simulink library "lib_controls"  (Simulink 7.9)
settings: Solver=ode45  SolverMode=SingleTasking  StartTime=0.0  StopTime=10.0  RelTol=1e-3
undefined symbols (not defined in the file or in its folder): amb_tmp, cs_charge_deplete_bool, cs_charge_pwr, cs_charge_trq, cs_clt_tmp, cs_decel_fc_off, cs_decel_regen_threshold, cs_dl_assist_trq_threshold, cs_dl_regen_trq_threshold, cs_electric_decel_spd, cs_electric_launch_spd, cs_electric_launch_spd_hi, cs_electric_launch_spd_lo, cs_eng_min_spd, cs_eng_on_soc, cs_fc_init_state, cs_fc_max_pwr_frac, cs_fc_min_pwr_frac, cs_fc_on, cs_fc_pwr_opt, cs_fc_spd_opt, cs_fuzzy_fuel_mode, cs_hi_soc, cs_hi_trq_frac, cs_lo_soc, cs_lo_trq_frac, cs_max_gc_spd, cs_max_pwr, cs_max_pwr_fall_rate, cs_max_pwr_rise_rate, cs_mc_assist_max_frac, cs_mc_assist_min_frac, cs_mc_assist_slope, cs_mc_regen_max_frac, cs_mc_regen_min_frac, cs_mc_regen_slope, cs_mean_eff, cs_mean_eff_bool, cs_min_gc_spd, cs_min_off_time, cs_min_pwr, cs_min_trq_frac, cs_mph_avg_time, cs_off_trq_frac, cs_plot_output, cs_pwr, cs_regen_avg_time, cs_scale_factor, cs_shutoff, cs_soc_range, cs_spd, cs_target_soc, cs_trq_to_soc_factor, cvt_locus_pwr, cvt_locus_spd, cyc_mph, enable_sim_stop_distance, enable_sim_stop_max_spd, enable_sim_stop_speed, enable_sim_stop_time ... (+110)
libraries: lib_controls x124, simulink3 x13, simulink x5, lib_etc x1
(part 2 of 17)

== system lib_controls/<vc> insight ==
  Ground : Ground
  Relational Operator : RelationalOperator  Operator=~=  InputSameDT=on
  Sum : Sum  Inputs=-+  SaturateOnIntegerOverflow=on  InputSameDT=on  OutDataTypeStr=Inherit: Same as first input
  braking strategy : lib_controls/SubSystem/braking strategy
  config traction control : Subsystem  BlockChoice=traction control 2 axle
      settings: AttributesFormatString=%<BlockChoice>  TemplateBlock=lib_controls/SubSystem/config traction control  MemberBlocks=traction control 2 axle,traction control J2452 2 axle
  engine on (insight) : Subsystem
  front and rear brake controller (achievable) : lib_controls/SubSystem/front and rear brake controller (achievable)
  motor controller logic : Subsystem
  parallel clutch control : Subsystem
  pre-TX parallel gearbox control : Subsystem
  sim stop subsystem : lib_controls/SubSystem/sim stop subsystem
  clutch state : Outport
  tag scope: F_front_brake=global, F_front_brake_req=global, F_rear_brake=global, F_rear_brake_req=global, F_req_limited=global, P_mc_in_r=global, clutch_state=global, engine_on=global, front_traction_ratio=global, gear_number=global, gear_ratio=global, key_on=global, shifting=global, slip_limited=global, spd_command=global, v_req_limited=global, wt_front_axle=global, wt_rear_axle=global
  wires:
  [eta_gb] -> pre-TX parallel gearbox control/3(prev. Pout/Pin)
  [w_gb_out] -> pre-TX parallel gearbox control/2(gb_spd_out_r)
  [T_gb_out] -> pre-TX parallel gearbox control/1(gb_trq_out_r)
  [slip_limited] -> pre-TX parallel gearbox control/4(tires are at traction limit)
  motor controller logic/1(req'd input power (W)1) -> [P_mc_in_r]
  [w_mc_out_r] -> motor controller logic/3(req'd output spd (rad/s))
  [P_mc_in_1lim] -> motor controller logic/2(req'd input power (W))
  [bus_voltage] -> motor controller logic/1(bus voltage)
  front and rear brake controller (achievable)/2 -> [F_rear_brake]
  [F_max_rear_brake] -> front and rear brake controller (achievable)/5
  [F_max_front_brake] -> front and rear brake controller (achievable)/4
  [w_wheel_ach] -> front and rear brake controller (achievable)/3
  [F_drivetrain_ach] -> front and rear brake controller (achievable)/2
  front and rear brake controller (achievable)/1 -> [F_front_brake]
  [v_ave_req] -> braking strategy/1, engine on (insight)/4(v_ave_req), config traction control/1(time-average vehicle speed  req'd (m/s))
  config traction control/3(weight on front axle (N)) -> [wt_front_axle]
  [v_prev] -> config traction control/2(vehicle speed at beginning of time  step (m/s))
  braking strategy/1 -> [F_front_brake_req]
  [F_req] -> front and rear brake controller (achievable)/1, Relational Operator/2, config traction control/3(total tractive force req'd (N))
  config traction control/1(req'd force (N)) -> braking strategy/2, Sum/2, Relational Operator/1
  braking strategy/2 -> Sum/1, [F_rear_brake_req]
  Sum/1 -> [F_req_limited]
  Relational Operator/1 -> [slip_limited]
  config traction control/2(req'd speed (m/s)) -> [v_req_limited]
  [shifting] -> motor controller logic/4(shifting)
  parallel clutch control/1(clutch state) -> [clutch_state], clutch state/1, engine on (insight)/5(clutch state)
  engine on (insight)/1(engine on) -> [engine_on], parallel clutch control/4(engine on)
  [w_cl_out] -> parallel clutch control/3(gb_spd_in_r), engine on (insight)/2(spd_clutch_out)
  engine on (insight)/2(spd command  (rad/s)) -> [spd_command]
  [fc_spd_out_r] -> engine on (insight)/3(fc_spd_out_r)
  engine on (insight)/3(key on) -> [key_on]
  [T_cl_out] -> parallel clutch control/2(gb_trq_in_r), engine on (insight)/1(trq_clutch_out)
  [shifting] -> parallel clutch control/1(shifting)
  pre-TX parallel gearbox control/3("shifting, out") -> [shifting]
  pre-TX parallel gearbox control/2("gear ratio, out") -> [gear_ratio]
  pre-TX parallel gearbox control/1("gear number, out") -> [gear_number]
  config traction control/4(weight on rear axle (N)) -> [wt_rear_axle]
  config traction control/5(front/total  traction ratio) -> [front_traction_ratio]
  Ground/1 -> front and rear brake controller (achievable)/6

== system lib_controls/<vc> par ==
  note: force
      | required (N)
  Ground : Ground
  Relational Operator : RelationalOperator  Operator=~=  InputSameDT=on
  Sum : Sum  Inputs=-+  SaturateOnIntegerOverflow=on  InputSameDT=on  OutDataTypeStr=Inherit: Same as first input
  braking strategy : lib_controls/SubSystem/braking strategy
  config traction control : Subsystem  BlockChoice=traction control 2 axle
      settings: AttributesFormatString=%<BlockChoice>  TemplateBlock=lib_controls/SubSystem/config traction control  MemberBlocks=traction control 2 axle,traction control J2452 2 axle
  engine on (parallel hybrid) : Subsystem
  front and rear brake controller (achievable) : lib_controls/SubSystem/front and rear brake controller (achievable)
  motor controller logic : Subsystem
  parallel clutch control : Subsystem
  pre-TX parallel gearbox control : Subsystem
  sim stop subsystem : lib_controls/SubSystem/sim stop subsystem
  clutch state : Outport
  tag scope: F_front_brake=global, F_front_brake_req=global, F_rear_brake=global, F_rear_brake_req=global, F_req_limited=global, P_mc_in_r=global, clutch_state=global, engine_on=global, front_traction_ratio=global, gear_number=global, gear_ratio=global, key_on=global, shifting=global, slip_limited=global, spd_command=global, v_req_limited=global, wt_front_axle=global, wt_rear_axle=global
  wires:
  [bus_voltage] -> motor controller logic/1(bus voltage)
  [P_mc_in_1lim] -> motor controller logic/2(req'd input power (W))
  [w_mc_out_r] -> motor controller logic/3(req'd output spd (rad/s))
  motor controller logic/1(req'd input power (W)1) -> [P_mc_in_r]
  [shifting] -> motor controller logic/4(shifting)
  [slip_limited] -> pre-TX parallel gearbox control/4(tires are at traction limit)
  [T_gb_out] -> pre-TX parallel gearbox control/1(gb_trq_out_r)
  [w_gb_out] -> pre-TX parallel gearbox control/2(gb_spd_out_r)
  [eta_gb] -> pre-TX parallel gearbox control/3(prev. Pout/Pin)
  engine on (parallel hybrid)/3(key on) -> [key_on]
  [fc_spd_out_r] -> engine on (parallel hybrid)/3(fc_spd_out_r)
  engine on (parallel hybrid)/2(spd command  (rad/s)) -> [spd_command]
  [v_ave_req] -> engine on (parallel hybrid)/4(v_ave_req)
  [w_cl_out] -> engine on (parallel hybrid)/2(spd req'd out of clutch (N*m)1)
  [T_cl_out] -> engine on (parallel hybrid)/1(trq req'd out of clutch (N*m))
  engine on (parallel hybrid)/1(engine on) -> [engine_on]
  [clutch_state] -> engine on (parallel hybrid)/5(clutch state)
  braking strategy/2 -> Sum/1, [F_rear_brake_req]
  config traction control/1(req'd force (N)) -> braking strategy/2, Sum/2, Relational Operator/1
  braking strategy/1 -> [F_front_brake_req]
  [v_prev] -> config traction control/2(vehicle speed at beginning of time  step (m/s))
  config traction control/2(req'd speed (m/s)) -> [v_req_limited]
  config traction control/3(weight on front axle (N)) -> [wt_front_axle]
  [F_req] -> config traction control/3(total tractive force req'd (N))
  Sum/1 -> [F_req_limited]
  [shifting] -> parallel clutch control/1(shifting)
  [w_cl_out] -> parallel clutch control/3(gb_spd_in_r)
  [T_cl_out] -> parallel clutch control/2(gb_trq_in_r)
  [engine_on] -> parallel clutch control/4(engine on)
  parallel clutch control/1(clutch state) -> [clutch_state], clutch state/1
  Relational Operator/1 -> [slip_limited]
  [F_req] -> Relational Operator/2
  [v_ave_req] -> config traction control/1(time-average vehicle speed  req'd (m/s))
  [v_ave_req] -> braking strategy/1
  front and rear brake controller (achievable)/1 -> [F_front_brake]
  [F_drivetrain_ach] -> front and rear brake controller (achievable)/2
  [w_wheel_ach] -> front and rear brake controller (achievable)/3
  [F_max_front_brake] -> front and rear brake controller (achievable)/4
  [F_max_rear_brake] -> front and rear brake controller (achievable)/5
  front and rear brake controller (achievable)/2 -> [F_rear_brake]
  [F_req] -> front and rear brake controller (achievable)/1
  pre-TX parallel gearbox control/1("gear number, out") -> [gear_number]
  pre-TX parallel gearbox control/2("gear ratio, out") -> [gear_ratio]
  pre-TX parallel gearbox control/3("shifting, out") -> [shifting]
  config traction control/4(weight on rear axle (N)) -> [wt_rear_axle]
  config traction control/5(front/total  traction ratio) -> [front_traction_ratio]
  Ground/1 -> front and rear brake controller (achievable)/6

== system lib_controls/<vc> par Adaptive ==
  Ground : Ground
  Relational Operator : RelationalOperator  Operator=~=  InputSameDT=on
  Sum : Sum  Inputs=-+  SaturateOnIntegerOverflow=on  InputSameDT=on  OutDataTypeStr=Inherit: Same as first input
  braking strategy : lib_controls/SubSystem/braking strategy
  config traction control : Subsystem  BlockChoice=traction control 2 axle
      settings: AttributesFormatString=%<BlockChoice>  TemplateBlock=lib_controls/SubSystem/config traction control  MemberBlocks=traction control 2 axle,traction control J2452 2 axle
  engine on (Adaptive) : Subsystem
  front and rear brake controller (achievable) : lib_controls/SubSystem/front and rear brake controller (achievable)
  motor controller logic : Subsystem
  parallel clutch control : Subsystem
  pre-TX parallel gearbox control : Subsystem
  sim stop subsystem : lib_controls/SubSystem/sim stop subsystem
  clutch state : Outport
  tag scope: F_front_brake=global, F_front_brake_req=global, F_rear_brake=global, F_rear_brake_req=global, F_req_limited=global, P_mc_in_r=global, clutch_state=global, engine_on=global, front_traction_ratio=global, gear_number=global, gear_ratio=global, shifting=global, slip_limited=global, v_req_limited=global, wt_front_axle=global, wt_rear_axle=global
  wires:
  [fc_trq_out_r] -> engine on (Adaptive)/1(trq req'd of engine)
  engine on (Adaptive)/1(engine on) -> [engine_on]
  motor controller logic/1(req'd input power (W)1) -> [P_mc_in_r]
  [w_mc_out_r] -> motor controller logic/3(req'd output spd (rad/s))
  [P_mc_in_1lim] -> motor controller logic/2(req'd input power (W))
  [bus_voltage] -> motor controller logic/1(bus voltage)
  [shifting] -> motor controller logic/4(shifting)
  [eta_gb] -> pre-TX parallel gearbox control/3(prev. Pout/Pin)
  [w_gb_out] -> pre-TX parallel gearbox control/2(gb_spd_out_r)
  [T_gb_out] -> pre-TX parallel gearbox control/1(gb_trq_out_r)
  [slip_limited] -> pre-TX parallel gearbox control/4(tires are at traction limit)
  config traction control/3(weight on front axle (N)) -> [wt_front_axle]
  config traction control/2(req'd speed (m/s)) -> [v_req_limited]
  [v_prev] -> config traction control/2(vehicle speed at beginning of time  step (m/s))
  braking strategy/1 -> [F_front_brake_req]
  config traction control/1(req'd force (N)) -> braking strategy/2, Sum/2, Relational Operator/1
  braking strategy/2 -> Sum/1, [F_rear_brake_req]
  parallel clutch control/1(clutch state) -> [clutch_state], clutch state/1
  [w_cl_out] -> parallel clutch control/3(gb_spd_in_r)
  [T_cl_out] -> parallel clutch control/2(gb_trq_in_r)
  [engine_on] -> parallel clutch control/4(engine on)
  [shifting] -> parallel clutch control/1(shifting)
  Sum/1 -> [F_req_limited]
  Relational Operator/1 -> [slip_limited]
  [F_req] -> Relational Operator/2
  [F_req] -> config traction control/3(total tractive force req'd (N))
  [v_ave_req] -> config traction control/1(time-average vehicle speed  req'd (m/s))
  [v_ave_req] -> braking strategy/1
  front and rear brake controller (achievable)/2 -> [F_rear_brake]
  [F_max_rear_brake] -> front and rear brake controller (achievable)/5
  [F_max_front_brake] -> front and rear brake controller (achievable)/4
  [w_wheel_ach] -> front and rear brake controller (achievable)/3
  [F_drivetrain_ach] -> front and rear brake controller (achievable)/2
  front and rear brake controller (achievable)/1 -> [F_front_brake]
  [F_req] -> front and rear brake controller (achievable)/1
  pre-TX parallel gearbox control/1("gear number, out") -> [gear_number]
  pre-TX parallel gearbox control/2("gear ratio, out") -> [gear_ratio]
  pre-TX parallel gearbox control/3("shifting, out") -> [shifting]
  config traction control/4(weight on rear axle (N)) -> [wt_rear_axle]
  config traction control/5(front/total  traction ratio) -> [front_traction_ratio]
  Ground/1 -> front and rear brake controller (achievable)/6

== system lib_controls/<vc> par auto ==
  Ground : Ground
  Relational Operator : RelationalOperator  Operator=~=  InputSameDT=on
  Sum : Sum  Inputs=-+  SaturateOnIntegerOverflow=on  InputSameDT=on  OutDataTypeStr=Inherit: Same as first input
  braking strategy : lib_controls/SubSystem/braking strategy
  config traction control : Subsystem  BlockChoice=traction control 2 axle
      settings: AttributesFormatString=%<BlockChoice>  TemplateBlock=lib_controls/SubSystem/config traction control  MemberBlocks=traction control 2 axle,traction control J2452 2 axle
  engine on (parallel hybrid) : Subsystem
  front and rear brake controller (achievable) : lib_controls/SubSystem/front and rear brake controller (achievable)
  gearbox control for use w/ AT : Subsystem
  motor controller logic : Subsystem
  parallel clutch control : Subsystem
  sim stop subsystem : lib_controls/SubSystem/sim stop subsystem
  clutch state : Outport
  tag scope: F_front_brake=global, F_front_brake_req=global, F_rear_brake=global, F_rear_brake_req=global, F_req_limited=global, P_mc_in_r=global, clutch_state=global, engine_on=global, front_traction_ratio=global, gear_number=global, gear_ratio=global, key_on=global, locked_up=global, shifting=global, slip_limited=global, spd_command=global, v_req_limited=global, wt_front_axle=global, wt_rear_axle=global
  wires:
  motor controller logic/1(req'd input power (W)1) -> [P_mc_in_r]
  [w_mc_out_r] -> motor controller logic/3(req'd output spd (rad/s))
  [P_mc_in_1lim] -> motor controller logic/2(req'd input power (W))
  [bus_voltage] -> motor controller logic/1(bus voltage)
  [shifting] -> motor controller logic/4(shifting)
  [eta_gb] -> gearbox control for use w/ AT/1(eta_gb)
  [T_gb_out] -> gearbox control for use w/ AT/2(gb_trq_out_r)
  [w_gb_out] -> gearbox control for use w/ AT/3(gb_spd_out_r)
  [slip_limited] -> gearbox control for use w/ AT/4(tires are at traction limit)
  gearbox control for use w/ AT/4(locked up) -> [locked_up]
  config traction control/3(weight on front axle (N)) -> [wt_front_axle]
  config traction control/2(req'd speed (m/s)) -> [v_req_limited]
  [v_prev] -> config traction control/2(vehicle speed at beginning of time  step (m/s))
  braking strategy/1 -> [F_front_brake_req]
  config traction control/1(req'd force (N)) -> braking strategy/2, Sum/2, Relational Operator/1
  [F_req] -> config traction control/3(total tractive force req'd (N))
  [v_ave_req] -> config traction control/1(time-average vehicle speed  req'd (m/s))
  [v_ave_req] -> braking strategy/1
  front and rear brake controller (achievable)/2 -> [F_rear_brake]
  [F_max_rear_brake] -> front and rear brake controller (achievable)/5
  [F_max_front_brake] -> front and rear brake controller (achievable)/4
  [w_wheel_ach] -> front and rear brake controller (achievable)/3
  [F_drivetrain_ach] -> front and rear brake controller (achievable)/2
  front and rear brake controller (achievable)/1 -> [F_front_brake]
  [F_req] -> front and rear brake controller (achievable)/1
  braking strategy/2 -> Sum/1, [F_rear_brake_req]
  Sum/1 -> [F_req_limited]
  Relational Operator/1 -> [slip_limited]
  [F_req] -> Relational Operator/2
  engine on (parallel hybrid)/2(spd command  (rad/s)) -> [spd_command]
  [fc_spd_out_r] -> engine on (parallel hybrid)/3(fc_spd_out_r)
  engine on (parallel hybrid)/3(key on) -> [key_on]
  [w_cl_out] -> engine on (parallel hybrid)/2(spd req'd out of clutch (N*m)1)
  [T_cl_out] -> engine on (parallel hybrid)/1(trq req'd out of clutch (N*m))
  engine on (parallel hybrid)/1(engine on) -> [engine_on]
  [v_ave_req] -> engine on (parallel hybrid)/4(v_ave_req)
  [clutch_state] -> engine on (parallel hybrid)/5(clutch state)
  parallel clutch control/1(clutch state) -> [clutch_state], clutch state/1
  [shifting] -> parallel clutch control/1(shifting)
  [w_cl_out] -> parallel clutch control/3(gb_spd_in_r)
  [T_cl_out] -> parallel clutch control/2(gb_trq_in_r)
  [engine_on] -> parallel clutch control/4(engine on)
  gearbox control for use w/ AT/1("gear number, out") -> [gear_number]
  gearbox control for use w/ AT/2("gear ratio, out") -> [gear_ratio]
  gearbox control for use w/ AT/3("shifting, out") -> [shifting]
  config traction control/4(weight on rear axle (N)) -> [wt_rear_axle]
  config traction control/5(front/total  traction ratio) -> [front_traction_ratio]
  Ground/1 -> front and rear brake controller (achievable)/6

== system lib_controls/<vc> par auto s/a ==
  note: force
      | required (N)
  Constant : Constant  Value=3
  Demux : Demux  Outputs=2
  Ground : Ground
  Relational Operator : RelationalOperator  Operator=~=  InputSameDT=on
  Sum : Sum  Inputs=-+  SaturateOnIntegerOverflow=on  InputSameDT=on  OutDataTypeStr=Inherit: Same as first input
  braking strategy : lib_controls/SubSystem/braking strategy
  config traction control : Subsystem  BlockChoice=traction control 2 axle
      settings: AttributesFormatString=%<BlockChoice>  TemplateBlock=lib_controls/SubSystem/config traction control  MemberBlocks=traction control 2 axle,traction control J2452 2 axle
  engine on (parallel hybrid) : Subsystem
  front and rear brake controller (achievable) : lib_controls/SubSystem/front and rear brake controller (achievable)
  gearbox control for use w/ AT  in parallel sa : Subsystem
  motor controller logic : Subsystem
  sim stop subsystem : lib_controls/SubSystem/sim stop subsystem
  tag scope: F_front_brake=global, F_front_brake_req=global, F_rear_brake=global, F_rear_brake_req=global, F_req_limited=global, P_mc_in_r=global, clutch_state=global, engine_on=global, front_traction_ratio=global, gear_number=global, gear_ratio=global, key_on=global, locked_up=global, shifting=global, slip_limited=global, spd_command=global, v_req_limited=global, wt_front_axle=global, wt_rear_axle=global
  wires:
  config traction control/1(req'd force (N)) -> braking strategy/2, Sum/2, Relational Operator/1
  braking strategy/1 -> [F_front_brake_req]
  [v_prev] -> config traction control/2(vehicle speed at beginning of time  step (m/s))
  config traction control/2(req'd speed (m/s)) -> [v_req_limited]
  config traction control/3(weight on front axle (N)) -> [wt_front_axle]
  Demux/1 -> engine on (parallel hybrid)/1(trq req'd out of clutch (N*m))
  [bus_voltage] -> motor controller logic/1(bus voltage)
  [P_mc_in_1lim] -> motor controller logic/2(req'd input power (W))
  [w_mc_out_r] -> motor controller logic/3(req'd output spd (rad/s))
  motor controller logic/1(req'd input power (W)1) -> [P_mc_in_r]
  [shifting] -> motor controller logic/4(shifting)
  Constant/1 -> [clutch_state]
  engine on (parallel hybrid)/3(key on) -> [key_on]
  [fc_spd_out_r] -> engine on (parallel hybrid)/3(fc_spd_out_r)
  engine on (parallel hybrid)/2(spd command  (rad/s)) -> [spd_command]
  engine on (parallel hybrid)/1(engine on) -> [engine_on]
  Demux/2 -> engine on (parallel hybrid)/2(spd req'd out of clutch (N*m)1)
  [v_ave_req] -> engine on (parallel hybrid)/4(v_ave_req)
  [tc_trq_spd_in_r] -> Demux/1
  [clutch_state] -> engine on (parallel hybrid)/5(clutch state)
  [slip_limited] -> gearbox control for use w/ AT  in parallel sa/4(tires are at traction limit)
  [w_gb_out] -> gearbox control for use w/ AT  in parallel sa/3(gb_spd_out_r)
  [T_gb_out] -> gearbox control for use w/ AT  in parallel sa/2(gb_trq_out_r)
  [eta_gb] -> gearbox control for use w/ AT  in parallel sa/1(eta_gb)
  [v_ave_req] -> config traction control/1(time-average vehicle speed  req'd (m/s))
  [v_ave_req] -> braking strategy/1
  [F_req] -> config traction control/3(total tractive force req'd (N))
  braking strategy/2 -> Sum/1, [F_rear_brake_req]
  Sum/1 -> [F_req_limited]
  Relational Operator/1 -> [slip_limited]
  [F_req] -> Relational Operator/2
  front and rear brake controller (achievable)/1 -> [F_front_brake]
  [F_drivetrain_ach] -> front and rear brake controller (achievable)/2
  [w_wheel_ach] -> front and rear brake controller (achievable)/3
  [F_max_front_brake] -> front and rear brake controller (achievable)/4
  [F_max_rear_brake] -> front and rear brake controller (achievable)/5
  front and rear brake controller (achievable)/2 -> [F_rear_brake]
  [F_req] -> front and rear brake controller (achievable)/1
  gearbox control for use w/ AT  in parallel sa/1("gear number, out") -> [gear_number]
  gearbox control for use w/ AT  in parallel sa/2("gear ratio, out") -> [gear_ratio]
  gearbox control for use w/ AT  in parallel sa/3("shifting, out") -> [shifting]
  gearbox control for use w/ AT  in parallel sa/4(locked up) -> [locked_up]
  config traction control/4(weight on rear axle (N)) -> [wt_rear_axle]
  config traction control/5(front/total  traction ratio) -> [front_traction_ratio]
  Ground/1 -> front and rear brake controller (achievable)/6

== system lib_controls/<vc> par balanced ==
  note: force
      | required (N)
  Ground : Ground
  Relational Operator : RelationalOperator  Operator=~=  InputSameDT=on
  Sum : Sum  Inputs=-+  SaturateOnIntegerOverflow=on  InputSameDT=on  OutDataTypeStr=Inherit: Same as first input
  braking strategy : lib_controls/SubSystem/braking strategy
  config traction control : Subsystem  BlockChoice=traction control 2 axle
      settings: AttributesFormatString=%<BlockChoice>  TemplateBlock=lib_controls/SubSystem/config traction control  MemberBlocks=traction control 2 axle,traction control J2452 2 axle
  engine on (balanced parallel hybrid) : Subsystem
  front and rear brake controller (achievable) : lib_controls/SubSystem/front and rear brake controller (achievable)
  motor controller logic : Subsystem
  parallel clutch control : Subsystem
  pre-TX parallel gearbox control : Subsystem
  sim stop subsystem : lib_controls/SubSystem/sim stop subsystem
  clutch state : Outport
  tag scope: F_front_brake=global, F_front_brake_req=global, F_rear_brake=global, F_rear_brake_req=global, F_req_limited=global, P_mc_in_r=global, clutch_state=global, engine_on=global, front_traction_ratio=global, gear_number=global, gear_ratio=global, key_on=global, shifting=global, slip_limited=global, spd_command=global, v_req_limited=global, wt_front_axle=global, wt_rear_axle=global
  wires:
  [bus_voltage] -> motor controller logic/1(bus voltage)
  [P_mc_in_1lim] -> motor controller logic/2(req'd input power (W))
  [w_mc_out_r] -> motor controller logic/3(req'd output spd (rad/s))
  motor controller logic/1(req'd input power (W)1) -> [P_mc_in_r]
  [shifting] -> motor controller logic/4(shifting)
  engine on (balanced parallel hybrid)/3(key on) -> [key_on]
  [fc_spd_out_r] -> engine on (balanced parallel hybrid)/3(fc_spd_out_r)
  engine on (balanced parallel hybrid)/2(spd command  (rad/s)) -> [spd_command]
  [clutch_state] -> engine on (balanced parallel hybrid)/5(clutch state)
  [v_ave_req] -> engine on (balanced parallel hybrid)/4(v_ave_req)
  [w_cl_out] -> engine on (balanced parallel hybrid)/2(spd req'd out of clutch (N*m)1)
  [T_cl_out] -> engine on (balanced parallel hybrid)/1(trq req'd out of clutch (N*m))
  engine on (balanced parallel hybrid)/1(engine on) -> [engine_on]
  parallel clutch control/1(clutch state) -> [clutch_state], clutch state/1
  [shifting] -> parallel clutch control/1(shifting)
  [w_cl_out] -> parallel clutch control/3(gb_spd_in_r)
  [T_cl_out] -> parallel clutch control/2(gb_trq_in_r)
  [engine_on] -> parallel clutch control/4(engine on)
  [slip_limited] -> pre-TX parallel gearbox control/4(tires are at traction limit)
  [T_gb_out] -> pre-TX parallel gearbox control/1(gb_trq_out_r)
  [w_gb_out] -> pre-TX parallel gearbox control/2(gb_spd_out_r)
  [eta_gb] -> pre-TX parallel gearbox control/3(prev. Pout/Pin)
  braking strategy/2 -> Sum/1, [F_rear_brake_req]
  config traction control/1(req'd force (N)) -> braking strategy/2, Sum/2, Relational Operator/1
  braking strategy/1 -> [F_front_brake_req]
  [v_prev] -> config traction control/2(vehicle speed at beginning of time  step (m/s))
  config traction control/2(req'd speed (m/s)) -> [v_req_limited]
  config traction control/3(weight on front axle (N)) -> [wt_front_axle]
  [v_ave_req] -> braking strategy/1
  [v_ave_req] -> config traction control/1(time-average vehicle speed  req'd (m/s))
  front and rear brake controller (achievable)/1 -> [F_front_brake]
  [F_drivetrain_ach] -> front and rear brake controller (achievable)/2
  [w_wheel_ach] -> front and rear brake controller (achievable)/3
  [F_max_front_brake] -> front and rear brake controller (achievable)/4
  [F_max_rear_brake] -> front and rear brake controller (achievable)/5
  front and rear brake controller (achievable)/2 -> [F_rear_brake]
  [F_req] -> front and rear brake controller (achievable)/1
  Sum/1 -> [F_req_limited]
  Relational Operator/1 -> [slip_limited]
  [F_req] -> config traction control/3(total tractive force req'd (N))
  [F_req] -> Relational Operator/2
  pre-TX parallel gearbox control/1("gear number, out") -> [gear_number]
  pre-TX parallel gearbox control/2("gear ratio, out") -> [gear_ratio]
  pre-TX parallel gearbox control/3("shifting, out") -> [shifting]
  config traction control/4(weight on rear axle (N)) -> [wt_rear_axle]
  config traction control/5(front/total  traction ratio) -> [front_traction_ratio]
  Ground/1 -> front and rear brake controller (achievable)/6

== system lib_controls/<vc> par cvt ==
  Constant2 : Constant  Value=0
  Ground : Ground
  Relational Operator : RelationalOperator  Operator=~=  InputSameDT=on
  Sum : Sum  Inputs=-+  SaturateOnIntegerOverflow=on  InputSameDT=on  OutDataTypeStr=Inherit: Same as first input
  braking strategy : lib_controls/SubSystem/braking strategy
  config traction control : Subsystem  BlockChoice=traction control 2 axle
      settings: AttributesFormatString=%<BlockChoice>  TemplateBlock=lib_controls/SubSystem/config traction control  MemberBlocks=traction control 2 axle,traction control J2452 2 axle
  cvt control : Subsystem
  engine on (parallel CVT hybrid) : Subsystem
  front and rear brake controller (achievable) : lib_controls/SubSystem/front and rear brake controller (achievable)
  motor controller logic : Subsystem
  parallel clutch control : Subsystem
  sim stop subsystem : lib_controls/SubSystem/sim stop subsystem
  clutch state : Outport
  tag scope: F_front_brake=global, F_front_brake_req=global, F_rear_brake=global, F_rear_brake_req=global, F_req_limited=global, P_mc_in_r=global, clutch_state=global, engine_on=global, front_traction_ratio=global, gear_ratio=global, key_on=global, shifting=global, slip_limited=global, spd_command=global, v_req_limited=global, wt_front_axle=global, wt_rear_axle=global
  wires:
  engine on (parallel CVT hybrid)/2(spd command  (rad/s)) -> [spd_command]
  [fc_spd_out_r] -> engine on (parallel CVT hybrid)/3(fc_spd_out_r)
  engine on (parallel CVT hybrid)/3(key on) -> [key_on]
  [clutch_state] -> engine on (parallel CVT hybrid)/5(clutch state)
  engine on (parallel CVT hybrid)/1(engine on) -> [engine_on]
  [T_cl_out] -> engine on (parallel CVT hybrid)/1(trq req'd out of clutch (N*m))
  [w_cl_out] -> engine on (parallel CVT hybrid)/2(spd req'd out of clutch (N*m)1)
  [v_ave_req] -> engine on (parallel CVT hybrid)/4(v_ave_req)
  parallel clutch control/1(clutch state) -> [clutch_state], clutch state/1
  [shifting] -> parallel clutch control/1(shifting)
  [engine_on] -> parallel clutch control/4(engine on)
  [T_cl_out] -> parallel clutch control/2(gb_trq_in_r)
  [w_cl_out] -> parallel clutch control/3(gb_spd_in_r)
  motor controller logic/1(req'd input power (W)1) -> [P_mc_in_r]
  [w_mc_out_r] -> motor controller logic/3(req'd output spd (rad/s))
  [P_mc_in_1lim] -> motor controller logic/2(req'd input power (W))
  [bus_voltage] -> motor controller logic/1(bus voltage)
  [shifting] -> motor controller logic/4(shifting)
  Constant2/1 -> [shifting]
  [T_gb_out] -> cvt control/1(cvt_trq_out_r)
  [eta_gb] -> cvt control/3(prev. Pout/Pin)
  [w_gb_out] -> cvt control/2(cvt_spd_out_r)
  [slip_limited] -> cvt control/4(tires are at traction limit)
  cvt control/1("pulley ratio ") -> [gear_ratio]
  config traction control/3(weight on front axle (N)) -> [wt_front_axle]
  config traction control/2(req'd speed (m/s)) -> [v_req_limited]
  [v_prev] -> config traction control/2(vehicle speed at beginning of time  step (m/s))
  braking strategy/1 -> [F_front_brake_req]
  config traction control/1(req'd force (N)) -> braking strategy/2, Sum/2, Relational Operator/1
  [F_req] -> config traction control/3(total tractive force req'd (N))
  braking strategy/2 -> Sum/1, [F_rear_brake_req]
  Sum/1 -> [F_req_limited]
  Relational Operator/1 -> [slip_limited]
  [F_req] -> Relational Operator/2
  [v_ave_req] -> config traction control/1(time-average vehicle speed  req'd (m/s))
  [v_ave_req] -> braking strategy/1
  front and rear brake controller (achievable)/2 -> [F_rear_brake]
  [F_max_rear_brake] -> front and rear brake controller (achievable)/5
  [F_max_front_brake] -> front and rear brake controller (achievable)/4
  [w_wheel_ach] -> front and rear brake controller (achievable)/3
  [F_drivetrain_ach] -> front and rear brake controller (achievable)/2
  front and rear brake controller (achievable)/1 -> [F_front_brake]
  [F_req] -> front and rear brake controller (achievable)/1
  config traction control/4(weight on rear axle (N)) -> [wt_rear_axle]
  config traction control/5(front/total  traction ratio) -> [front_traction_ratio]
  Ground/1 -> front and rear brake controller (achievable)/6

== system lib_controls/<vc> prius ==
  note: force required (N)
  Coordinated  Controller : Subsystem
  Ground : Ground
  Relational Operator : RelationalOperator  Operator=~=  InputSameDT=on
  Sum : Sum  Inputs=-+  SaturateOnIntegerOverflow=on  InputSameDT=on  OutDataTypeStr=Inherit: Same as first input
  braking strategy : lib_controls/SubSystem/braking strategy
  config traction control : Subsystem  BlockChoice=traction control 2 axle
      settings: AttributesFormatString=%<BlockChoice>  TemplateBlock=lib_controls/SubSystem/config traction control  MemberBlocks=traction control 2 axle,traction control J2452 2 axle
  front and rear brake controller (achievable) : lib_controls/SubSystem/front and rear brake controller (achievable)
  key_on : Subsystem  mask(Repeating table){t=vc_key_on(:,1), y=vc_key_on(:,2)}
      mask prompts: t "Time values:"; y "Output values:"
      mask help:
      | Repeating table.
      | Enter values of time and output for first cycle.
      mask init:
      | period = max(t);
      mask Help: Repeats cycle given in table. Time values should be monotonically increasing.
  prius generator  controller logic : Subsystem
  prius motor  controller logic : Subsystem
  sim stop subsystem : lib_controls/SubSystem/sim stop subsystem
  tag scope: F_front_brake=global, F_front_brake_req=global, F_rear_brake=global, F_rear_brake_req=global, F_req_limited=global, P_gc_in_r=global, P_mc_in_r=global, fc_spd_req=global, fc_trq_req=global, front_traction_ratio=global, key_on=global, slip_limited=global, v_req_limited=global, wt_front_axle=global, wt_rear_axle=global
  wires:
  prius motor  controller logic/1(req'd input power (W)1) -> [P_mc_in_r]
  [w_mc_out_r] -> prius motor  controller logic/3(req'd output spd (rad/s))
  [P_mc_in_1lim] -> prius motor  controller logic/2(req'd input power (W))
  [bus_voltage] -> prius motor  controller logic/1(bus voltage)
  prius generator  controller logic/1(req'd input power (W)1) -> [P_gc_in_r]
  [w_gc_out_r] -> prius generator  controller logic/3(req'd output spd (rad/s))
  [P_gc_in_1lim] -> prius generator  controller logic/2(req'd input power (W))
  [bus_voltage] -> prius generator  controller logic/1(bus voltage)
  [pgs_trq_spd_r] -> Coordinated  Controller/1("(Trq and speed req'd  from ring gear) Nm, rad/s")
  Coordinated  Controller/2(fc spd request) -> [fc_spd_req]
  [SOC] -> Coordinated  Controller/2(soc)
  Coordinated  Controller/1(fc trq request) -> [fc_trq_req]
  key_on/1(out_1) -> [key_on]
  config traction control/3(weight on front axle (N)) -> [wt_front_axle]
  config traction control/2(req'd speed (m/s)) -> [v_req_limited]
  [v_prev] -> config traction control/2(vehicle speed at beginning of time  step (m/s))
  braking strategy/1 -> [F_front_brake_req]
  config traction control/1(req'd force (N)) -> braking strategy/2, Sum/2, Relational Operator/1
  braking strategy/2 -> Sum/1, [F_rear_brake_req]
  Relational Operator/1 -> [slip_limited]
  Sum/1 -> [F_req_limited]
  [F_req] -> config traction control/3(total tractive force req'd (N))
  [v_ave_req] -> config traction control/1(time-average vehicle speed  req'd (m/s))
  [v_ave_req] -> braking strategy/1
  [F_req] -> Relational Operator/2
  front and rear brake controller (achievable)/2 -> [F_rear_brake]
  [F_max_rear_brake] -> front and rear brake controller (achievable)/5
  [F_max_front_brake] -> front and rear brake controller (achievable)/4
  [w_wheel_ach] -> front and rear brake controller (achievable)/3
  [F_drivetrain_ach] -> front and rear brake controller (achievable)/2
  front and rear brake controller (achievable)/1 -> [F_front_brake]
  [F_req] -> front and rear brake controller (achievable)/1
  config traction control/4(weight on rear axle (N)) -> [wt_rear_axle]
  config traction control/5(front/total  traction ratio) -> [front_traction_ratio]
  Ground/1 -> front and rear brake controller (achievable)/6

== system lib_controls/<vc> series ==
  Ground : Ground
  Relational Operator : RelationalOperator  Operator=~=  InputSameDT=on
  Sum : Sum  Inputs=-+  SaturateOnIntegerOverflow=on  InputSameDT=on  OutDataTypeStr=Inherit: Same as first input
  braking strategy : lib_controls/SubSystem/braking strategy
  config traction control : Subsystem  BlockChoice=traction control 2 axle
      settings: AttributesFormatString=%<BlockChoice>  TemplateBlock=lib_controls/SubSystem/config traction control  MemberBlocks=traction control 2 axle,traction control J2452 2 axle
  front and rear brake controller (achievable) : lib_controls/SubSystem/front and rear brake controller (achievable)
  gearbox control for series  HV and EV : Subsystem
  key_on : Subsystem  mask(Repeating table){t=vc_key_on(:,1), y=vc_key_on(:,2)}
      mask prompts: t "Time values:"; y "Output values:"
      mask help:
      | Repeating table.
      | Enter values of time and output for first cycle.
      mask init:
      | period = max(t);
      mask Help: Repeats cycle given in table. Time values should be monotonically increasing.
  motor controller logic : Subsystem
  series 'clutch' control : Subsystem
  sim stop subsystem : lib_controls/SubSystem/sim stop subsystem
  tag scope: F_front_brake=global, F_front_brake_req=global, F_rear_brake=global, F_rear_brake_req=global, F_req_limited=global, P_mc_in_r=global, clutch_state=global, front_traction_ratio=global, gear_number=global, gear_ratio=global, key_on=global, shifting=global, slip_limited=global, v_req_limited=global, wt_front_axle=global, wt_rear_axle=global
  wires:
  motor controller logic/1(req'd input power (W)1) -> [P_mc_in_r]
  [bus_voltage] -> motor controller logic/1(bus voltage)
  [P_mc_in_1lim] -> motor controller logic/2(req'd input power (W))
  [w_mc_out_r] -> motor controller logic/3(req'd output spd (rad/s))
  [shifting] -> motor controller logic/4(shifting)
  [eta_gb] -> gearbox control for series  HV and EV/3(prev. Pout/Pin)
  [w_gb_out] -> gearbox control for series  HV and EV/2(gb_spd_out_r)
  [T_gb_out] -> gearbox control for series  HV and EV/1(gb_trq_out_r)
  [slip_limited] -> gearbox control for series  HV and EV/4(tires are at traction limit)
  series 'clutch' control/1(clutch state) -> [clutch_state]
  [engine_on] -> series 'clutch' control/1(engine on)
  key_on/1(out_1) -> [key_on]
  front and rear brake controller (achievable)/1 -> [F_front_brake]
  [F_drivetrain_ach] -> front and rear brake controller (achievable)/2
  [w_wheel_ach] -> front and rear brake controller (achievable)/3
  [F_max_front_brake] -> front and rear brake controller (achievable)/4
  [F_max_rear_brake] -> front and rear brake controller (achievable)/5
  front and rear brake controller (achievable)/2 -> [F_rear_brake]
  [F_req] -> front and rear brake controller (achievable)/1
  braking strategy/1 -> [F_front_brake_req]
  [v_ave_req] -> braking strategy/1
  braking strategy/2 -> Sum/1, [F_rear_brake_req]
  config traction control/1(req'd force (N)) -> braking strategy/2, Sum/2, Relational Operator/1
  [v_prev] -> config traction control/2(vehicle speed at beginning of time  step (m/s))
  config traction control/2(req'd speed (m/s)) -> [v_req_limited]
  config traction control/3(weight on front axle (N)) -> [wt_front_axle]
  [F_req] -> config traction control/3(total tractive force req'd (N))
  Sum/1 -> [F_req_limited]
  Relational Operator/1 -> [slip_limited]
  [F_req] -> Relational Operator/2
  [v_ave_req] -> config traction control/1(time-average vehicle speed  req'd (m/s))
  gearbox control for series  HV and EV/3("shifting, out") -> [shifting]
  gearbox control for series  HV and EV/2("gear ratio, out") -> [gear_ratio]
  gearbox control for series  HV and EV/1("gear number, out") -> [gear_number]
  config traction control/4(weight on rear axle (N)) -> [wt_rear_axle]
  config traction control/5(front/total  traction ratio) -> [front_traction_ratio]
  Ground/1 -> front and rear brake controller (achievable)/6

== system lib_controls/Adaptive control strategy <cs> ==
  "trq and spd req'd into clutch (N*m, rad/s)" : Inport
  Delta SOC expected from regen : Subsystem
  Finds operation  point - energy/emissions  weighting : Subsystem
  Mux1 : Mux  Inputs=2
  spd : Selector  InputPortWidth=2  IndexOptions=Index vector (dialog)  Indices=2  OutputSizes=1
  "trq and spd req'd from engine (N*m, rad/s)" : Outport
  tag scope: fc_trq_out_r=global
  wires:
  Mux1/1 -> "trq and spd req'd from engine (N*m, rad/s)"/1
  spd/1 -> Mux1/2
  Delta SOC expected from regen/1(Delta SOC regen) -> Finds operation  point - energy/emissions  weighting/2(Delta SOC expected from regen)
  "trq and spd req'd into clutch (N*m, rad/s)"/1 -> spd/1, Finds operation  point - energy/emissions  weighting/1("trq and spd req'd into clutch (N*m, rad/s)"), Delta SOC expected from regen/1("trq and spd req'd into clutch (N*m, rad/s)")
  Finds operation  point - energy/emissions  weighting/1(trq req'd from  engine (N*m)) -> Mux1/1, [fc_trq_out_r]

== system lib_controls/Fuzzy Logic control strategy <cs> ==
  note: FUZZY CONTROL BLOCK
  note: Speed is directly fed through
  "trq and spd req'd into clutch (N*m, rad/s)" : Inport
  Block NOTES : Subsystem
      mask Display: disp('Block\nNOTES')
  Demux : Demux  Outputs=2
  Fuzzy logic Code : Subsystem
  Input Scaling : Subsystem
  Mux : Mux  Inputs=2
  Output scaling : Subsystem
  To Workspace4 : ToWorkspace  VariableName=cs_trq_in_r  SampleTime=-1
  To Workspace5 : ToWorkspace  VariableName=cs_spd_in_r  SampleTime=-1
  help : Subsystem
      settings: OpenFcn=web(['file:\\\' which('fuzzy_logic.htm')]);
      mask Display: image(imread('doc_man.jpg'))
  "trq and spd req'd from engine (N*m, rad/s)" : Outport
  wires:
  Output scaling/1(ICE Torque command) -> Mux/1
  Mux/1 -> "trq and spd req'd from engine (N*m, rad/s)"/1
  Fuzzy logic Code/1(delta  alpha) -> Output scaling/1("delta alpha ")
  Input Scaling/1(Torque) -> Fuzzy logic Code/1(Torque)
  Input Scaling/2(SoC) -> Fuzzy logic Code/2(SoC)
  "trq and spd req'd into clutch (N*m, rad/s)"/1 -> Demux/1
  Demux/2 -> To Workspace5/1, Mux/2
  Demux/1 -> To Workspace4/1, Input Scaling/1(Torque required)

== system lib_controls/Fuzzy Logic control strategy with Emissions <cs> ==
  note: FUZZY CONTROL BLOCK
  note: Speed is directly fed through
  "trq and spd req'd into clutch (N*m, rad/s)" : Inport
  Block NOTES : Subsystem
      mask Display: disp('Block\nNOTES')
  Demux : Demux  Outputs=2
  Fuzzy logic Code : Subsystem
  Input Scaling : Subsystem
  Mux : Mux  Inputs=2
  Output scaling : Subsystem
  "SoC " : Subsystem
  To Workspace4 : ToWorkspace  VariableName=cs_trq_in_r  SampleTime=-1
  To Workspace5 : ToWorkspace  VariableName=cs_spd_in_r  SampleTime=-1
  "trq and spd req'd from engine (N*m, rad/s)" : Outport
  wires:
  Fuzzy logic Code/1(delta  alpha) -> Output scaling/1("delta alpha ")
  Input Scaling/1(Torque) -> Fuzzy logic Code/1(Torque)
  "trq and spd req'd into clutch (N*m, rad/s)"/1 -> Demux/1
  Demux/2 -> To Workspace5/1, Mux/2
  Demux/1 -> To Workspace4/1, Input Scaling/1(Torque required)
  Mux/1 -> "trq and spd req'd from engine (N*m, rad/s)"/1
  "SoC "/1(SoC) -> Fuzzy logic Code/2(SoC)
  Output scaling/1(ICE Torque command) -> Mux/1

== system lib_controls/Insight electric assist control strategy <cs> DIRECT SPLIT ==
  note: ICE Torque
  note: Total Torque
  note: EM Torque
  note: Speed is directly fed through
  note: Motor Spins at ICE speed
  note: HONDA INSIGHT CONTROL STRATEGY
  "trq and spd req'd into clutch (N*m, rad/s)" : Inport
  1st gear ? : Subsystem
  Alternator Function : Subsystem
  Block NOTES : Subsystem
      mask Display: disp('Block\nNOTES')
  Clutch Engaged ? : Subsystem
  Constant7 : Constant  Value=0
  Demux : Demux  Outputs=2
  Hard Acceleration : Subsystem
  Hard Deceleration : Subsystem
  Mux : Mux  Inputs=2
  Mux1 : Mux  Inputs=2
  No EM activity at Slow Speed : Subsystem
  SoC Correction : Subsystem
  Sum : Sum  Inputs=-+  SaturateOnIntegerOverflow=on  InputSameDT=on  OutDataTypeStr=Inherit: Same as first input
  Switch7 : Switch  Threshold=eps  SaturateOnIntegerOverflow=on  InputSameDT=on
  To Workspace2 : ToWorkspace  VariableName=cs_trq_in_r  SampleTime=-1
  To Workspace3 : ToWorkspace  VariableName=cs_spd_in_r  SampleTime=-1
  help : Subsystem
      settings: OpenFcn=web(['file:\\\' which('honda_insight.htm')]);
      mask Display: image(imread('doc_man.jpg'))
  "trq and spd req'd from engine (N*m, rad/s)" : Outport
  "trq and spd req'd from MOTOR (N*m, rad/s)" : Outport  Port=2
  tag scope: cs_trq_in_r=global
  wires:
  Hard Deceleration/1(Out1) -> 1st gear ?/2(In 2), Hard Acceleration/2(In2)
  "trq and spd req'd into clutch (N*m, rad/s)"/1 -> Demux/1
  Demux/2 -> To Workspace3/1, Alternator Function/2(In2), Mux/2
  Demux/1 -> To Workspace2/1, Sum/2, Hard Deceleration/1(In1), Hard Acceleration/1(In1), [cs_trq_in_r]
  Hard Acceleration/1(Out1) -> 1st gear ?/1(In 1)
  Sum/1 -> Switch7/1
  Constant7/1 -> Switch7/3
  [engine_on] -> Switch7/2
  Mux/1 -> "trq and spd req'd from engine (N*m, rad/s)"/1
  Switch7/1 -> Mux/1
  Mux1/1 -> "trq and spd req'd from MOTOR (N*m, rad/s)"/1
  Alternator Function/1(Motor torque) -> Clutch Engaged ?/1(In1)
  1st gear ?/1(Out1) -> No EM activity at Slow Speed/1(In1)
  No EM activity at Slow Speed/1(Out1) -> Alternator Function/1(In1)
  Alternator Function/2(alternator torque) -> Clutch Engaged ?/2(In2)
  [spd_command] -> Mux1/2
  Clutch Engaged ?/1(Out1) -> SoC Correction/1(In1)
  SoC Correction/1(Out1) -> Sum/1, Mux1/1

== system lib_controls/SubSystem ==
  note: required
      | force (N)
  note: required force
      | (from traction control)
  note: required rear
      | brake force
  note: SUB MODEL LIBRARY FOR VEHICLE CONTROLS
  note: this shifting block part
      | of the speed dependent
      |  shifting above
  Speed Dependent Shifting : Subsystem
  braking strategy : Subsystem
  config traction control : Subsystem  BlockChoice=traction control 2 axle
      settings: TemplateBlock=self  MemberBlocks=traction control 2 axle,traction control J2452 2 axle
  current veh mass (kg) : Subsystem
  front and rear brake controller (achievable) : Subsystem
  shifting : Subsystem
  sim stop subsystem : Subsystem
  traction control : Subsystem
  traction control 2 axle : Subsystem
  traction control J2452 : Subsystem  AncestorBlock="lib_controls/SubSystem/traction  control"
  traction control J2452 2 axle : Subsystem
  tag scope: F_front_brake=global, F_front_brake_req=global, F_rear_brake=global, v_req_limited=global, wt_front_axle=global
  wires:
  [v_ave_req] -> traction control/1(time-average vehicle speed  req'd (m/s))
  [v_prev] -> traction control/2(vehicle speed at beginning of time  step (m/s))
  [F_req] -> traction control/3(total tractive force req'd (N))
  traction control/3(weight on front axle (N)) -> [wt_front_axle]
  traction control/2(req'd speed (m/s)) -> [v_req_limited]
  [v_ave_req] -> braking strategy/1(req'd speed (m/s))
  braking strategy/1(req'd front brake force (N)) -> [F_front_brake_req]
  [F_req] -> front and rear brake controller (achievable)/1(total tractive force req'd (N))
  [F_drivetrain_ach] -> front and rear brake controller (achievable)/2(tractive force available from  front drivetrain (N))
  [w_wheel_ach] -> front and rear brake controller (achievable)/3(axle speed possible (rad/s))
  [F_max_front_brake] -> front and rear brake controller (achievable)/4(max front brake force (N))
  [F_max_rear_brake] -> front and rear brake controller (achievable)/5(max rear brake force (N))
  front and rear brake controller (achievable)/1(front-axle braking force (N)) -> [F_front_brake]
  front and rear brake controller (achievable)/2(rear-axle braking force (N)) -> [F_rear_brake]
  [v_req_limited] -> Speed Dependent Shifting/1("velocity required (limited) ")
  Speed Dependent Shifting/1(gear ratio and shifting) -> [spd_dep_muxed]
  Speed Dependent Shifting/2(gear number) -> [spd_dep_gear_num]
  [F_rear_drivetrain_ach] -> front and rear brake controller (achievable)/6(tractive force available from  rear drivetrain (N))

== system lib_controls/electric assist control strategy <cs> ==
  "trq and spd req'd into clutch (N*m, rad/s)" : Inport
  Constant : Constant  Value=0
  Demux : Demux  Outputs=2
  MinMax : MinMax  Function=max  Inputs=2  SaturateOnIntegerOverflow=on  InputSameDT=on
  Mux : Mux  Inputs=2
  Sum : Sum  SaturateOnIntegerOverflow=on  InputSameDT=on  OutDataTypeStr=Inherit: Same as first input
  Switch : Switch  Threshold=eps  SaturateOnIntegerOverflow=on  InputSameDT=on
  chg trq req'd (Nm) : Subsystem
  help : Subsystem
      settings: OpenFcn=web(['file:\\\' which('Parallel.htm')])
      mask Display: image(imread('doc_man.jpg'))
  minimum trq (Nm) : Subsystem
  "trq and spd req'd from engine (N*m, rad/s)" : Outport
  wires:
  "trq and spd req'd into clutch (N*m, rad/s)"/1 -> minimum trq (Nm)/1("trq and spd req'd into trq coupler (N*m, rad/s)"), Demux/1
  chg trq req'd (Nm)/1(add'l trq req'd (Nm)) -> Sum/1
  Sum/1 -> MinMax/1
  MinMax/1 -> Switch/1
  Constant/1 -> Switch/3
  Switch/1 -> Mux/1
  Mux/1 -> "trq and spd req'd from engine (N*m, rad/s)"/1
  Demux/2 -> Mux/2
  minimum trq (Nm)/1(minimum trq (N*m)) -> MinMax/2
  [engine_on] -> Switch/2
  Demux/1 -> Sum/2

== system lib_controls/electric assist control strategy bal <cs> ==
  "trq and spd req'd into clutch (N*m, rad/s)" : Inport
  Constant : Constant  Value=0
  MinMax : MinMax  Function=max  Inputs=2  SaturateOnIntegerOverflow=on  InputSameDT=on
  Mux : Mux  Inputs=2
  SOC corrected  trq req'd (N*m) : Subsystem
  Selector : Selector  InputPortWidth=2  IndexOptions=Index vector (dialog)  Indices=2  OutputSizes=1
  Switch : Switch  Threshold=eps  SaturateOnIntegerOverflow=on  InputSameDT=on
  help : Subsystem
      settings: OpenFcn=web(['file:\\\' which('Parallel.htm')])
      mask Display: image(imread('doc_man.jpg'))
  minimum trq (N*m) : Subsystem
  "trq and spd req'd from engine (N*m, rad/s)" : Outport
  wires:
  SOC corrected  trq req'd (N*m)/1(SOC corrected  trq req'd (N*m)) -> MinMax/1
  MinMax/1 -> Switch/1
  "trq and spd req'd into clutch (N*m, rad/s)"/1 -> SOC corrected  trq req'd (N*m)/1("trq and spd req'd into trq coupler (N*m, rad/s)"), Selector/1, minimum trq (N*m)/1("trq and spd req'd into trq coupler (N*m, rad/s)")
  minimum trq (N*m)/1(minimum trq (N*m)) -> MinMax/2
  [engine_on] -> Switch/2
  Selector/1 -> Mux/2
  Mux/1 -> "trq and spd req'd from engine (N*m, rad/s)"/1
  Switch/1 -> Mux/1
  Constant/1 -> Switch/3
